simulink model "CASE_i_12b"  (R2020a)
settings: Solver=ode45  StartTime=0.0  StopTime=60  RelTol=1e-3  EnableMultiTasking=on
libraries: simulink x1
settings Model: Creator=Prof Francisco M. Gonzalez-Longatt  LastModifiedBy=fglon
settings DataIOCC: LimitDataPoints=on  SaveFormat=Array  SignalLoggingSaveFormat=ModelDataLogs  ReturnWorkspaceOutputs=off  SignalLoggingName=sigsOut
settings DebuggingCC: SaveWithParameterizedLinksMsg=none  UnderspecifiedInitializationDetection=Classic  MergeDetectMultiDrivingBlocksExec=none  SignalResolutionControl=TryResolveAllWithWarning  MultiTaskDSMMsg=warning  MultiTaskCondExecSysMsg=none
settings HardwareCC: ProdBitPerPointer=32  ProdBitPerSizeT=32  ProdBitPerPtrDiffT=32  ProdLargestAtomicFloat=None  ProdIntDivRoundTo=Undefined  ProdEndianess=Unspecified  ProdWordSize=32  ProdHWDeviceType=32-bit Generic  TargetUnknown=on
settings ModelReferenceCC: PropagateSignalLabelsOutOfModel=off
settings GRTTargetCC: CombineOutputUpdateFcns=off  GRTInterface=on
settings ConfigComp: CovMetricSettings=dw  CovHtmlReporting=on  CovSaveCumulativeToWorkspaceVar=on  CovSaveSingleToWorkspaceVar=on

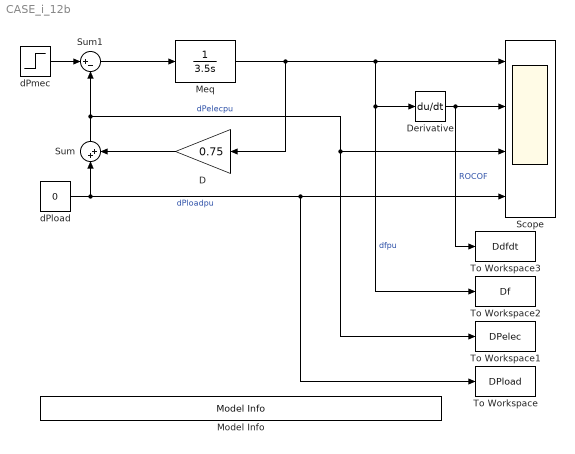
== system CASE_i_12b ==
  D : Gain  Gain=0.75  SaturateOnIntegerOverflow=on  OutDataTypeStr=Inherit: Same as input  ParamDataTypeStr=Inherit: Same as input
  Derivative : Derivative
  Meq : TransferFcn  Denominator=[3.5 0]
  Model Info : simulink/Model-Wide Utilities/Model Info  Frame=on  DisplayStringWithTags=|  HorizontalTextAlignment=Center  LeftAlignmentValue=0.5
      | Generator Outage in an Isolated Area
      | %<Creator>
  Scope : Scope  NumInputPorts=4
  Sum : Sum  Inputs=|++  SaturateOnIntegerOverflow=on
  Sum1 : Sum  Inputs=|+-  SaturateOnIntegerOverflow=on
  To Workspace : ToWorkspace  VariableName=DPload  SampleTime=-1
  To Workspace1 : ToWorkspace  VariableName=DPelec  SampleTime=-1
  To Workspace2 : ToWorkspace  VariableName=Df  SampleTime=-1
  To Workspace3 : ToWorkspace  VariableName=Ddfdt  SampleTime=-1
  dPload : Constant  Value=0
  dPmec : Step  Time=0  After=-0.375  SampleTime=0
  wires:
  Meq/1 -> D/1, Derivative/1, To Workspace2/1, Scope/1  "dfpu"
  D/1 -> Sum/2
  Sum1/1 -> Meq/1
  Sum/1 -> Sum1/2, Scope/3, To Workspace1/1  "dPelecpu"
  Derivative/1 -> Scope/2, To Workspace3/1  "ROCOF"
  dPload/1 -> Sum/1, Scope/4, To Workspace/1  "dPloadpu"
  dPmec/1 -> Sum1/1
